simulink library "halin"  (R2021b)
settings: Solver=VariableStepAuto  StartTime=0.0  StopTime=10.0  RelTol=1e-3
undefined symbols (not defined in the file): KHAL_CAN1ABM1E2E_flg, KHAL_CAN1EPB1E2E_flg, KHAL_CAN1EPS1E2E_flg, KHAL_CAN1ESC1E2E_flg, KHAL_CAN1ESC5E2E_flg, KHAL_CAN3BMS1E2E_flg, KHAL_CAN3BMS6E2E_flg, KHAL_CAN3CCU1E2E_flg, KHAL_CAN3CCU2E2E_flg, KHAL_CAN3MCUNF1E2E_flg, KHAL_CAN3MCUNR1E2E_flg, KHAL_CAN3Shifter1E2E_flg, KHAL_CAN3Shifter2E2E_flg, KHAL_CAN6FCM2E2E_flg, KHAL_CAN6FCM4E2E_flg, TRUE
libraries: simulink x645, FVT_lib x212, hcu_lib x59
(part 11 of 23)

== system halin/HAL_IN/CAN3/CCU1 ==
  DT_CAN3_SG_CCU1 : Inport
  0x35 : Constant  Value=0x35
  0xEB : Constant  Value=0xEB
  BitwiseAND{,1..24} (25 alike) : simulink/Logic and Bit Operations/Bitwise Operator  logicop=AND  UseBitMask=on  BitMask=0xFF  BitMaskRealWorld=Stored Integer
  BitwiseOR{,1..2,9..11} (6 alike) : simulink/Logic and Bit Operations/Bitwise Operator  logicop=OR  UseBitMask=off  BitMask=bin2dec('11011001')  BitMaskRealWorld=Stored Integer
  BitwiseOR3 : simulink/Logic and Bit Operations/Bitwise Operator  logicop=OR  UseBitMask=off  NumInputPorts=3  BitMask=bin2dec('11011001')  BitMaskRealWorld=Stored Integer
  BitwiseOR4 : simulink/Logic and Bit Operations/Bitwise Operator  logicop=OR  UseBitMask=off  NumInputPorts=2  BitMask=bin2dec('11011001')  BitMaskRealWorld=Stored Integer
  BitwiseOR5 : simulink/Logic and Bit Operations/Bitwise Operator  logicop=OR  UseBitMask=off  NumInputPorts=3  BitMask=bin2dec('11011001')  BitMaskRealWorld=Stored Integer
  BitwiseOR6 : simulink/Logic and Bit Operations/Bitwise Operator  logicop=OR  UseBitMask=off  NumInputPorts=2  BitMask=bin2dec('11011001')  BitMaskRealWorld=Stored Integer
  BitwiseOR7 : simulink/Logic and Bit Operations/Bitwise Operator  logicop=OR  UseBitMask=off  NumInputPorts=2  BitMask=bin2dec('11011001')  BitMaskRealWorld=Stored Integer
  BitwiseOR8 : simulink/Logic and Bit Operations/Bitwise Operator  logicop=OR  UseBitMask=off  NumInputPorts=7  BitMask=bin2dec('11011001')  BitMaskRealWorld=Stored Integer
  CSCCU1 : Subsystem
  DCDCAuxCur : Subsystem
  DCDCAuxVolt : Subsystem
  DCDCHVCur : Subsystem
  DCDCInVoltInf : Subsystem
  DCDCPreCompleted : Subsystem
  DDM_CS&RC_Comparison : FVT_lib/hal/DDM_CS&RC_Comparison  MsgCycleTime=10
  Data Type Conversion{,1..24} (25 alike) : DataTypeConversion  OutDataTypeStr=uint8
  KHAL_CAN3CCU1E2E_flg : Constant  Value=KHAL_CAN3CCU1E2E_flg
  LeftShift : ArithShift  BitShiftDirection=Left
  LeftShift1 : ArithShift  BitShiftNumber=5  BitShiftDirection=Left
  LeftShift10 : ArithShift  BitShiftDirection=Left
  LeftShift2 : ArithShift  BitShiftNumber=4  BitShiftDirection=Left
  LeftShift3 : ArithShift  BitShiftNumber=5  BitShiftDirection=Left
  LeftShift4 : ArithShift  BitShiftNumber=3  BitShiftDirection=Left
  LeftShift5 : ArithShift  BitShiftNumber=2  BitShiftDirection=Left
  LeftShift6 : ArithShift  BitShiftNumber=6  BitShiftDirection=Left
  LeftShift7 : ArithShift  BitShiftNumber=7  BitShiftDirection=Left
  LeftShift8 : ArithShift  BitShiftDirection=Left
  LeftShift9 : ArithShift  BitShiftNumber=3  BitShiftDirection=Left
  MessageRollingCounter : FVT_lib/hal/MessageRollingCounter  CounterMAX=14  task_time_ms=5  msg_time_ms=10
  Mux : Mux  Inputs=11
  OBCDCCurrInf : Subsystem
  OBCDCVoltInf : Subsystem
  OBCPreCompleted : Subsystem
  OBCWakeup4Plugin : Subsystem
  RCCCU1 : Subsystem
  RightShift : ArithShift  BitShiftNumber=4
  RightShift1 : ArithShift  BitShiftNumber=-4
  RightShift10 : ArithShift  BitShiftNumber=4
  RightShift11 : ArithShift  BitShiftNumber=-4
  RightShift12 : ArithShift  BitShiftNumber=1
  RightShift13 : ArithShift  BitShiftNumber=-7
  RightShift2 : ArithShift  BitShiftNumber=7
  RightShift3 : ArithShift  BitShiftNumber=-1
  RightShift4 : ArithShift  BitShiftNumber=8
  RightShift5 : ArithShift
  RightShift6 : ArithShift  BitShiftNumber=7
  RightShift7 : ArithShift  BitShiftNumber=-1
  RightShift8 : ArithShift  BitShiftNumber=7
  RightShift9 : ArithShift  BitShiftNumber=-1
  bus_selector : BusSelector  OutputSignals=CAN3_CS_CCU1,CAN3_DCDCAuxCur,CAN3_DCDCAuxVolt,CAN3_DCDCHVCur,CAN3_DCDCInVoltInf,CAN3_DCDCPreCompleted,CAN3_OBCDCCurrInf,CAN3_OBCDCVoltInf,CAN3_OBCPreCompleted,CAN3_OBCV2LINVOTP,CAN3_OBCV2LInsuFault,CAN3_OBCV2LVinOVP,CAN3_OBCV2LVinUVP,CAN3_OBCV2LVoutOCP,CAN3_OBCV2LVoutOVP,CAN3_OBCV2LVoutUVP,CAN3_OBCWakeup4Plugin,CAN3_RC_CCU1
  bus_selector1 : BusSelector  OutputSignals=CAN3_CS_CCU1
  bus_selector10 : BusSelector  OutputSignals=CAN3_OBCWakeup4Plugin
  bus_selector11 : BusSelector  OutputSignals=CAN3_RC_CCU1
  bus_selector2 : BusSelector  OutputSignals=CAN3_DCDCAuxCur
  bus_selector3 : BusSelector  OutputSignals=CAN3_DCDCAuxVolt
  bus_selector4 : BusSelector  OutputSignals=CAN3_DCDCHVCur
  bus_selector5 : BusSelector  OutputSignals=CAN3_DCDCInVoltInf
  bus_selector6 : BusSelector  OutputSignals=CAN3_DCDCPreCompleted
  bus_selector7 : BusSelector  OutputSignals=CAN3_OBCDCCurrInf
  bus_selector8 : BusSelector  OutputSignals=CAN3_OBCDCVoltInf
  bus_selector9 : BusSelector  OutputSignals=CAN3_OBCPreCompleted
  VHAL_CCU1CSErr_flg : Outport
  VHAL_CCU1RCErr_flg : Outport  Port=2
  VHAL_CSCCU1_enum : Outport  Port=3
  VHAL_DCDCAuxCur_A : Outport  Port=4
  VHAL_DCDCAuxVolt_V : Outport  Port=5
  VHAL_DCDCHVCur_A : Outport  Port=6
  VHAL_DCDCInVoltInf_V : Outport  Port=7
  VHAL_DCDCPreCompleted_enum : Outport  Port=8
  VHAL_OBCDCCurrInf_A : Outport  Port=9
  VHAL_OBCDCVoltInf_V : Outport  Port=10
  VHAL_OBCPreCompleted_enum : Outport  Port=11
  VHAL_OBCWakeup4Plugin_flg : Outport  Port=12
  VHAL_RCCCU1_enum : Outport  Port=13
  wires:
  DT_CAN3_SG_CCU1/1 -> [DT_CAN3_SG_CCU1]
  [DT_CAN3_SG_CCU1] -> bus_selector/1
  bus_selector/1 -> [CAN3_CS_CCU1]  "<CAN3_CS_CCU1>"
  [CAN3_CS_CCU1] -> LeftShift/1
  LeftShift/1 -> BitwiseAND/1
  BitwiseAND/1 -> [Byte_0_CAN3_CS_CCU1]
  bus_selector/2 -> [CAN3_DCDCAuxCur]  "<CAN3_DCDCAuxCur>"
  [CAN3_DCDCAuxCur] -> RightShift/1, RightShift1/1
  RightShift/1 -> BitwiseAND1/1
  BitwiseAND1/1 -> [Byte_10_CAN3_DCDCAuxCur]
  RightShift1/1 -> BitwiseAND2/1
  BitwiseAND2/1 -> [Byte_11_CAN3_DCDCAuxCur]
  bus_selector/3 -> [CAN3_DCDCAuxVolt]  "<CAN3_DCDCAuxVolt>"
  [CAN3_DCDCAuxVolt] -> RightShift2/1, RightShift3/1
  RightShift2/1 -> BitwiseAND3/1
  BitwiseAND3/1 -> [Byte_6_CAN3_DCDCAuxVolt]
  RightShift3/1 -> BitwiseAND4/1
  BitwiseAND4/1 -> [Byte_7_CAN3_DCDCAuxVolt]
  bus_selector/4 -> [CAN3_DCDCHVCur]  "<CAN3_DCDCHVCur>"
  [CAN3_DCDCHVCur] -> RightShift4/1, RightShift5/1
  RightShift4/1 -> BitwiseAND5/1
  BitwiseAND5/1 -> [Byte_8_CAN3_DCDCHVCur]
  RightShift5/1 -> BitwiseAND6/1
  BitwiseAND6/1 -> [Byte_9_CAN3_DCDCHVCur]
  bus_selector/5 -> [CAN3_DCDCInVoltInf]  "<CAN3_DCDCInVoltInf>"
  [CAN3_DCDCInVoltInf] -> RightShift6/1, RightShift7/1
  RightShift6/1 -> BitwiseAND7/1
  BitwiseAND7/1 -> [Byte_5_CAN3_DCDCInVoltInf]
  RightShift7/1 -> BitwiseAND8/1
  BitwiseAND8/1 -> [Byte_6_CAN3_DCDCInVoltInf]
  bus_selector/6 -> [CAN3_DCDCPreCompleted]  "<CAN3_DCDCPreCompleted>"
  [CAN3_DCDCPreCompleted] -> LeftShift1/1
  LeftShift1/1 -> BitwiseAND9/1
  BitwiseAND9/1 -> [Byte_5_CAN3_DCDCPreCompleted]
  bus_selector/7 -> [CAN3_OBCDCCurrInf]  "<CAN3_OBCDCCurrInf>"
  [CAN3_OBCDCCurrInf] -> RightShift8/1, RightShift9/1
  RightShift8/1 -> BitwiseAND10/1
  BitwiseAND10/1 -> [Byte_3_CAN3_OBCDCCurrInf]
  RightShift9/1 -> BitwiseAND11/1
  BitwiseAND11/1 -> [Byte_4_CAN3_OBCDCCurrInf]
  bus_selector/8 -> [CAN3_OBCDCVoltInf]  "<CAN3_OBCDCVoltInf>"
  [CAN3_OBCDCVoltInf] -> RightShift10/1, RightShift11/1
  RightShift10/1 -> BitwiseAND12/1
  BitwiseAND12/1 -> [Byte_2_CAN3_OBCDCVoltInf]
  RightShift11/1 -> BitwiseAND13/1
  BitwiseAND13/1 -> [Byte_3_CAN3_OBCDCVoltInf]
  bus_selector/9 -> [CAN3_OBCPreCompleted]  "<CAN3_OBCPreCompleted>"
  [CAN3_OBCPreCompleted] -> RightShift12/1, RightShift13/1
  RightShift12/1 -> BitwiseAND14/1
  BitwiseAND14/1 -> [Byte_4_CAN3_OBCPreCompleted]
  RightShift13/1 -> BitwiseAND15/1
  BitwiseAND15/1 -> [Byte_5_CAN3_OBCPreCompleted]
  bus_selector/10 -> [CAN3_OBCV2LINVOTP]  "<CAN3_OBCV2LINVOTP>"
  [CAN3_OBCV2LINVOTP] -> LeftShift2/1
  LeftShift2/1 -> BitwiseAND16/1
  BitwiseAND16/1 -> [Byte_8_CAN3_OBCV2LINVOTP]
  bus_selector/11 -> [CAN3_OBCV2LInsuFault]  "<CAN3_OBCV2LInsuFault>"
  [CAN3_OBCV2LInsuFault] -> LeftShift3/1
  LeftShift3/1 -> BitwiseAND17/1
  BitwiseAND17/1 -> [Byte_8_CAN3_OBCV2LInsuFault]
  bus_selector/12 -> [CAN3_OBCV2LVinOVP]  "<CAN3_OBCV2LVinOVP>"
  [CAN3_OBCV2LVinOVP] -> LeftShift4/1
  LeftShift4/1 -> BitwiseAND18/1
  BitwiseAND18/1 -> [Byte_8_CAN3_OBCV2LVinOVP]
  bus_selector/13 -> [CAN3_OBCV2LVinUVP]  "<CAN3_OBCV2LVinUVP>"
  [CAN3_OBCV2LVinUVP] -> LeftShift5/1
  LeftShift5/1 -> BitwiseAND19/1
  BitwiseAND19/1 -> [Byte_8_CAN3_OBCV2LVinUVP]
  bus_selector/14 -> [CAN3_OBCV2LVoutOCP]  "<CAN3_OBCV2LVoutOCP>"
  [CAN3_OBCV2LVoutOCP] -> LeftShift6/1
  LeftShift6/1 -> BitwiseAND20/1
  BitwiseAND20/1 -> [Byte_8_CAN3_OBCV2LVoutOCP]
  bus_selector/15 -> [CAN3_OBCV2LVoutOVP]  "<CAN3_OBCV2LVoutOVP>"
  [CAN3_OBCV2LVoutOVP] -> LeftShift7/1
  LeftShift7/1 -> BitwiseAND21/1
  BitwiseAND21/1 -> [Byte_8_CAN3_OBCV2LVoutOVP]
  bus_selector/16 -> [CAN3_OBCV2LVoutUVP]  "<CAN3_OBCV2LVoutUVP>"
  [CAN3_OBCV2LVoutUVP] -> LeftShift8/1
  LeftShift8/1 -> BitwiseAND22/1
  BitwiseAND22/1 -> [Byte_7_CAN3_OBCV2LVoutUVP]
  bus_selector/17 -> [CAN3_OBCWakeup4Plugin]  "<CAN3_OBCWakeup4Plugin>"
  [CAN3_OBCWakeup4Plugin] -> LeftShift9/1
  LeftShift9/1 -> BitwiseAND23/1
  BitwiseAND23/1 -> [Byte_3_CAN3_OBCWakeup4Plugin]
  bus_selector/18 -> [CAN3_RC_CCU1]  "<CAN3_RC_CCU1>"
  [CAN3_RC_CCU1] -> LeftShift10/1
  LeftShift10/1 -> BitwiseAND24/1
  BitwiseAND24/1 -> [Byte_1_CAN3_RC_CCU1]
  Data Type Conversion/1 -> BitwiseOR/1
  [Byte_0_CAN3_CS_CCU1] -> Data Type Conversion/1
  BitwiseOR/1 -> [Byte_0]
  Data Type Conversion1/1 -> BitwiseOR1/1
  [Byte_1_CAN3_RC_CCU1] -> Data Type Conversion1/1
  BitwiseOR1/1 -> [Byte_1]
  Data Type Conversion2/1 -> BitwiseOR2/1
  [Byte_2_CAN3_OBCDCVoltInf] -> Data Type Conversion2/1
  BitwiseOR2/1 -> [Byte_2]
  Data Type Conversion3/1 -> BitwiseOR3/1
  [Byte_3_CAN3_OBCDCCurrInf] -> Data Type Conversion3/1
  Data Type Conversion4/1 -> BitwiseOR3/2
  [Byte_3_CAN3_OBCDCVoltInf] -> Data Type Conversion4/1
  Data Type Conversion5/1 -> BitwiseOR3/3
  [Byte_3_CAN3_OBCWakeup4Plugin] -> Data Type Conversion5/1
  BitwiseOR3/1 -> [Byte_3]
  Data Type Conversion6/1 -> BitwiseOR4/1
  [Byte_4_CAN3_OBCDCCurrInf] -> Data Type Conversion6/1
  Data Type Conversion7/1 -> BitwiseOR4/2
  [Byte_4_CAN3_OBCPreCompleted] -> Data Type Conversion7/1
  BitwiseOR4/1 -> [Byte_4]
  Data Type Conversion8/1 -> BitwiseOR5/1
  [Byte_5_CAN3_DCDCInVoltInf] -> Data Type Conversion8/1
  Data Type Conversion9/1 -> BitwiseOR5/2
  [Byte_5_CAN3_DCDCPreCompleted] -> Data Type Conversion9/1
  Data Type Conversion10/1 -> BitwiseOR5/3
  [Byte_5_CAN3_OBCPreCompleted] -> Data Type Conversion10/1
  BitwiseOR5/1 -> [Byte_5]
  Data Type Conversion11/1 -> BitwiseOR6/1
  [Byte_6_CAN3_DCDCAuxVolt] -> Data Type Conversion11/1
  Data Type Conversion12/1 -> BitwiseOR6/2
  [Byte_6_CAN3_DCDCInVoltInf] -> Data Type Conversion12/1
  BitwiseOR6/1 -> [Byte_6]
  Data Type Conversion13/1 -> BitwiseOR7/1
  [Byte_7_CAN3_DCDCAuxVolt] -> Data Type Conversion13/1
  Data Type Conversion14/1 -> BitwiseOR7/2
  [Byte_7_CAN3_OBCV2LVoutUVP] -> Data Type Conversion14/1
  BitwiseOR7/1 -> [Byte_7]
  Data Type Conversion15/1 -> BitwiseOR8/1
  [Byte_8_CAN3_DCDCHVCur] -> Data Type Conversion15/1
  Data Type Conversion16/1 -> BitwiseOR8/2
  [Byte_8_CAN3_OBCV2LINVOTP] -> Data Type Conversion16/1
  Data Type Conversion17/1 -> BitwiseOR8/3
  [Byte_8_CAN3_OBCV2LInsuFault] -> Data Type Conversion17/1
  Data Type Conversion18/1 -> BitwiseOR8/4
  [Byte_8_CAN3_OBCV2LVinOVP] -> Data Type Conversion18/1
  Data Type Conversion19/1 -> BitwiseOR8/5
  [Byte_8_CAN3_OBCV2LVinUVP] -> Data Type Conversion19/1
  Data Type Conversion20/1 -> BitwiseOR8/6
  [Byte_8_CAN3_OBCV2LVoutOCP] -> Data Type Conversion20/1
  Data Type Conversion21/1 -> BitwiseOR8/7
  [Byte_8_CAN3_OBCV2LVoutOVP] -> Data Type Conversion21/1
  BitwiseOR8/1 -> [Byte_8]
  Data Type Conversion22/1 -> BitwiseOR9/1
  [Byte_9_CAN3_DCDCHVCur] -> Data Type Conversion22/1
  BitwiseOR9/1 -> [Byte_9]
  Data Type Conversion23/1 -> BitwiseOR10/1
  [Byte_10_CAN3_DCDCAuxCur] -> Data Type Conversion23/1
  BitwiseOR10/1 -> [Byte_10]
  Data Type Conversion24/1 -> BitwiseOR11/1
  [Byte_11_CAN3_DCDCAuxCur] -> Data Type Conversion24/1
  BitwiseOR11/1 -> [Byte_11]
  [Byte_1] -> Mux/1
  [Byte_2] -> Mux/2
  [Byte_3] -> Mux/3
  [Byte_4] -> Mux/4
  [Byte_5] -> Mux/5
  [Byte_6] -> Mux/6
  [Byte_7] -> Mux/7
  [Byte_8] -> Mux/8
  [Byte_9] -> Mux/9
  [Byte_10] -> Mux/10
  [Byte_11] -> Mux/11
  Mux/1 -> [VHAL_CAN3CCU1noCS_raw]
  KHAL_CAN3CCU1E2E_flg/1 -> DDM_CS&RC_Comparison/1
  0x35/1 -> DDM_CS&RC_Comparison/2
  0xEB/1 -> DDM_CS&RC_Comparison/3
  [VHAL_CAN3CCU1noCS_raw] -> DDM_CS&RC_Comparison/4
  [Byte_0] -> DDM_CS&RC_Comparison/5
  [RC_ECU] -> DDM_CS&RC_Comparison/6
  MessageRollingCounter/1 -> DDM_CS&RC_Comparison/7
  DDM_CS&RC_Comparison/1 -> VHAL_CCU1CSErr_flg/1
  DDM_CS&RC_Comparison/2 -> VHAL_CCU1RCErr_flg/1
  [DT_CAN3_SG_CCU1] -> bus_selector1/1
  bus_selector1/1 -> CSCCU1/1(CS_CCU1)  "<CAN3_CS_CCU1>"
  CSCCU1/1(VHAL_CSCCU1_enum) -> VHAL_CSCCU1_enum/1
  [DT_CAN3_SG_CCU1] -> bus_selector2/1
  bus_selector2/1 -> DCDCAuxCur/1(DCDCAuxCur)  "<CAN3_DCDCAuxCur>"
  DCDCAuxCur/1(VHAL_DCDCAuxCur_A) -> VHAL_DCDCAuxCur_A/1
  [DT_CAN3_SG_CCU1] -> bus_selector3/1
  bus_selector3/1 -> DCDCAuxVolt/1(DCDCAuxVolt)  "<CAN3_DCDCAuxVolt>"
  DCDCAuxVolt/1(VHAL_DCDCAuxVolt_V) -> VHAL_DCDCAuxVolt_V/1
  [DT_CAN3_SG_CCU1] -> bus_selector4/1
  bus_selector4/1 -> DCDCHVCur/1(DCDCHVCur)  "<CAN3_DCDCHVCur>"
  DCDCHVCur/1(VHAL_DCDCHVCur_A) -> VHAL_DCDCHVCur_A/1
  [DT_CAN3_SG_CCU1] -> bus_selector5/1
  bus_selector5/1 -> DCDCInVoltInf/1(DCDCInVoltInf)  "<CAN3_DCDCInVoltInf>"
  DCDCInVoltInf/1(VHAL_DCDCInVoltInf_V) -> VHAL_DCDCInVoltInf_V/1
  [DT_CAN3_SG_CCU1] -> bus_selector6/1
  bus_selector6/1 -> DCDCPreCompleted/1(DCDCPreCompleted)  "<CAN3_DCDCPreCompleted>"
  DCDCPreCompleted/1(VHAL_DCDCPreCompleted_enum) -> VHAL_DCDCPreCompleted_enum/1
  [DT_CAN3_SG_CCU1] -> bus_selector7/1
  bus_selector7/1 -> OBCDCCurrInf/1(OBCDCCurrInf)  "<CAN3_OBCDCCurrInf>"
  OBCDCCurrInf/1(VHAL_OBCDCCurrInf_A) -> VHAL_OBCDCCurrInf_A/1
  [DT_CAN3_SG_CCU1] -> bus_selector8/1
  bus_selector8/1 -> OBCDCVoltInf/1(OBCDCVoltInf)  "<CAN3_OBCDCVoltInf>"
  OBCDCVoltInf/1(VHAL_OBCDCVoltInf_V) -> VHAL_OBCDCVoltInf_V/1
  [DT_CAN3_SG_CCU1] -> bus_selector9/1
  bus_selector9/1 -> OBCPreCompleted/1(OBCPreCompleted)  "<CAN3_OBCPreCompleted>"
  OBCPreCompleted/1(VHAL_OBCPreCompleted_enum) -> VHAL_OBCPreCompleted_enum/1
  [DT_CAN3_SG_CCU1] -> bus_selector10/1
  bus_selector10/1 -> OBCWakeup4Plugin/1(OBCWakeup4Plugin)  "<CAN3_OBCWakeup4Plugin>"
  OBCWakeup4Plugin/1(VHAL_OBCWakeup4Plugin_flg) -> VHAL_OBCWakeup4Plugin_flg/1
  [DT_CAN3_SG_CCU1] -> bus_selector11/1
  bus_selector11/1 -> RCCCU1/1(RC_CCU1)  "<CAN3_RC_CCU1>"
  RCCCU1/1(VHAL_RCCCU1_enum) -> VHAL_RCCCU1_enum/1, [RC_ECU]

== system halin/HAL_IN/CAN3/CCU2 ==
  DT_CAN3_SG_CCU2 : Inport
  0x21 : Constant  Value=0x21
  0xE6 : Constant  Value=0xE6
  BitwiseAND{,1..20} (21 alike) : simulink/Logic and Bit Operations/Bitwise Operator  logicop=AND  UseBitMask=on  BitMask=0xFF  BitMaskRealWorld=Stored Integer
  BitwiseOR{,1..2,4..5,7..9} (8 alike) : simulink/Logic and Bit Operations/Bitwise Operator  logicop=OR  UseBitMask=off  BitMask=bin2dec('11011001')  BitMaskRealWorld=Stored Integer
  BitwiseOR10 : simulink/Logic and Bit Operations/Bitwise Operator  logicop=OR  UseBitMask=off  NumInputPorts=5  BitMask=bin2dec('11011001')  BitMaskRealWorld=Stored Integer
  BitwiseOR3 : simulink/Logic and Bit Operations/Bitwise Operator  logicop=OR  UseBitMask=off  NumInputPorts=3  BitMask=bin2dec('11011001')  BitMaskRealWorld=Stored Integer
  BitwiseOR6 : simulink/Logic and Bit Operations/Bitwise Operator  logicop=OR  UseBitMask=off  NumInputPorts=5  BitMask=bin2dec('11011001')  BitMaskRealWorld=Stored Integer
  CSCCU2 : Subsystem
  DCDCEnaSta : Subsystem
  DCDCFaultSta : Subsystem
  DCDCReady4Pre : Subsystem
  DCDCTemp : Subsystem
  DDM_CS&RC_Comparison : FVT_lib/hal/DDM_CS&RC_Comparison  MsgCycleTime=100
  Data Type Conversion{,1..20} (21 alike) : DataTypeConversion  OutDataTypeStr=uint8
  KHAL_CAN3CCU2E2E_flg : Constant  Value=KHAL_CAN3CCU2E2E_flg
  LeftShift{,4,6,12} (4 alike) : ArithShift  BitShiftDirection=Left
  LeftShift1 : ArithShift  BitShiftNumber=2  BitShiftDirection=Left
  LeftShift10 : ArithShift  BitShiftNumber=6  BitShiftDirection=Left
  LeftShift11 : ArithShift  BitShiftNumber=4  BitShiftDirection=Left
  LeftShift2 : ArithShift  BitShiftNumber=2  BitShiftDirection=Left
  LeftShift3 : ArithShift  BitShiftNumber=5  BitShiftDirection=Left
  LeftShift5 : ArithShift  BitShiftNumber=4  BitShiftDirection=Left
  LeftShift7 : ArithShift  BitShiftNumber=3  BitShiftDirection=Left
  LeftShift8 : ArithShift  BitShiftNumber=4  BitShiftDirection=Left
  LeftShift9 : ArithShift  BitShiftNumber=6  BitShiftDirection=Left
  MessageRollingCounter : FVT_lib/hal/MessageRollingCounter  CounterMAX=14  task_time_ms=5  msg_time_ms=100
  Mux : Mux  Inputs=11
  OBCACCurLim : Subsystem
  OBCACCurrInf : Subsystem
  OBCACVoltInf : Subsystem
  OBCEnaSta : Subsystem
  OBCFaultSta : Subsystem
  OBCPluginSta : Subsystem
  OBCReady4Pre : Subsystem
  OBCTemp : Subsystem
  OBCV2LSta : Subsystem
  RCCCU2 : Subsystem
  RightShift : ArithShift  BitShiftNumber=2
  RightShift1 : ArithShift  BitShiftNumber=-6
  RightShift2 : ArithShift  BitShiftNumber=8
  RightShift3 : ArithShift
  RightShift4 : ArithShift  BitShiftNumber=8
  RightShift5 : ArithShift
  RightShift6 : ArithShift  BitShiftNumber=1
  RightShift7 : ArithShift  BitShiftNumber=-7
  bus_selector : BusSelector  OutputSignals=CAN3_CS_CCU2,CAN3_DCDCEnaSta,CAN3_DCDCFaultSta,CAN3_DCDCReady4Pre,CAN3_DCDCTemp,CAN3_OBCACCurrInf,CAN3_OBCACVoltInf,CAN3_OBCDCP,CAN3_OBCEnaSta,CAN3_OBCFaultSta,CAN3_OBCPluginSta,CAN3_OBCReady4Pre,CAN3_OBCRlySta,CAN3_OBCTemp,CAN3_OBCV2LSta,CAN3_OBC_AC_Cur_Lim,CAN3_RC_CCU2
  bus_selector1 : BusSelector  OutputSignals=CAN3_CS_CCU2
  bus_selector10 : BusSelector  OutputSignals=CAN3_OBCPluginSta
  bus_selector11 : BusSelector  OutputSignals=CAN3_OBCReady4Pre
  bus_selector12 : BusSelector  OutputSignals=CAN3_OBCTemp
  bus_selector13 : BusSelector  OutputSignals=CAN3_OBCV2LSta
  bus_selector14 : BusSelector  OutputSignals=CAN3_OBC_AC_Cur_Lim
  bus_selector15 : BusSelector  OutputSignals=CAN3_RC_CCU2
  bus_selector2 : BusSelector  OutputSignals=CAN3_DCDCEnaSta
  bus_selector3 : BusSelector  OutputSignals=CAN3_DCDCFaultSta
  bus_selector4 : BusSelector  OutputSignals=CAN3_DCDCReady4Pre
  bus_selector5 : BusSelector  OutputSignals=CAN3_DCDCTemp
  bus_selector6 : BusSelector  OutputSignals=CAN3_OBCACCurrInf
  bus_selector7 : BusSelector  OutputSignals=CAN3_OBCACVoltInf
  bus_selector8 : BusSelector  OutputSignals=CAN3_OBCEnaSta
  bus_selector9 : BusSelector  OutputSignals=CAN3_OBCFaultSta
  constant : Constant  Value=0x0  OutDataTypeStr=uint8
  VHAL_CCU2CSErr_flg : Outport
  VHAL_CCU2RCErr_flg : Outport  Port=2
  VHAL_CSCCU2_enum : Outport  Port=3
  VHAL_DCDCEnaSta_flg : Outport  Port=4
  VHAL_DCDCFaultSta_enum : Outport  Port=5
  VHAL_DCDCReady4Pre_flg : Outport  Port=6
  VHAL_DCDCTemp_C : Outport  Port=7
  VHAL_OBCACCurrInf_A : Outport  Port=8
  VHAL_OBCACVoltInf_V : Outport  Port=9
  VHAL_OBCEnaSta_flg : Outport  Port=10
  VHAL_OBCFaultSta_enum : Outport  Port=11
  VHAL_OBCPluginSta_flg : Outport  Port=12
  VHAL_OBCReady4Pre_flg : Outport  Port=13
  VHAL_OBCTemp_C : Outport  Port=14
  VHAL_OBCV2LSta_enum : Outport  Port=15
  VHAL_OBCACCurLim_enum : Outport  Port=16
  VHAL_RCCCU2_enum : Outport  Port=17
  wires:
  DT_CAN3_SG_CCU2/1 -> [DT_CAN3_SG_CCU2]
  [DT_CAN3_SG_CCU2] -> bus_selector/1
  bus_selector/1 -> [CAN3_CS_CCU2]  "<CAN3_CS_CCU2>"
  [CAN3_CS_CCU2] -> LeftShift/1
  LeftShift/1 -> BitwiseAND/1
  BitwiseAND/1 -> [Byte_0_CAN3_CS_CCU2]
  bus_selector/2 -> [CAN3_DCDCEnaSta]  "<CAN3_DCDCEnaSta>"
  [CAN3_DCDCEnaSta] -> LeftShift1/1
  LeftShift1/1 -> BitwiseAND1/1
  BitwiseAND1/1 -> [Byte_7_CAN3_DCDCEnaSta]
  bus_selector/3 -> [CAN3_DCDCFaultSta]  "<CAN3_DCDCFaultSta>"
  [CAN3_DCDCFaultSta] -> LeftShift2/1
  LeftShift2/1 -> BitwiseAND2/1
  BitwiseAND2/1 -> [Byte_11_CAN3_DCDCFaultSta]
  bus_selector/4 -> [CAN3_DCDCReady4Pre]  "<CAN3_DCDCReady4Pre>"
  [CAN3_DCDCReady4Pre] -> LeftShift3/1
  LeftShift3/1 -> BitwiseAND3/1
  BitwiseAND3/1 -> [Byte_11_CAN3_DCDCReady4Pre]
  bus_selector/5 -> [CAN3_DCDCTemp]  "<CAN3_DCDCTemp>"
  [CAN3_DCDCTemp] -> LeftShift4/1
  LeftShift4/1 -> BitwiseAND4/1
  BitwiseAND4/1 -> [Byte_9_CAN3_DCDCTemp]
  bus_selector/6 -> [CAN3_OBCACCurrInf]  "<CAN3_OBCACCurrInf>"
  [CAN3_OBCACCurrInf] -> RightShift/1, RightShift1/1
  RightShift/1 -> BitwiseAND5/1
  BitwiseAND5/1 -> [Byte_6_CAN3_OBCACCurrInf]
  RightShift1/1 -> BitwiseAND6/1
  BitwiseAND6/1 -> [Byte_7_CAN3_OBCACCurrInf]
  bus_selector/7 -> [CAN3_OBCACVoltInf]  "<CAN3_OBCACVoltInf>"
  [CAN3_OBCACVoltInf] -> RightShift2/1, RightShift3/1
  RightShift2/1 -> BitwiseAND7/1
  BitwiseAND7/1 -> [Byte_4_CAN3_OBCACVoltInf]
  RightShift3/1 -> BitwiseAND8/1
  BitwiseAND8/1 -> [Byte_5_CAN3_OBCACVoltInf]
  bus_selector/8 -> [CAN3_OBCDCP]  "<CAN3_OBCDCP>"
  [CAN3_OBCDCP] -> RightShift4/1, RightShift5/1
  RightShift4/1 -> BitwiseAND9/1
  BitwiseAND9/1 -> [Byte_7_CAN3_OBCDCP]
  RightShift5/1 -> BitwiseAND10/1
  BitwiseAND10/1 -> [Byte_8_CAN3_OBCDCP]
  bus_selector/9 -> [CAN3_OBCEnaSta]  "<CAN3_OBCEnaSta>"
  [CAN3_OBCEnaSta] -> LeftShift5/1
  LeftShift5/1 -> BitwiseAND11/1
  BitwiseAND11/1 -> [Byte_7_CAN3_OBCEnaSta]
  bus_selector/10 -> [CAN3_OBCFaultSta]  "<CAN3_OBCFaultSta>"
  [CAN3_OBCFaultSta] -> LeftShift6/1
  LeftShift6/1 -> BitwiseAND12/1
  BitwiseAND12/1 -> [Byte_11_CAN3_OBCFaultSta]
  bus_selector/11 -> [CAN3_OBCPluginSta]  "<CAN3_OBCPluginSta>"
  [CAN3_OBCPluginSta] -> LeftShift7/1
  LeftShift7/1 -> BitwiseAND13/1
  BitwiseAND13/1 -> [Byte_7_CAN3_OBCPluginSta]
  bus_selector/12 -> [CAN3_OBCReady4Pre]  "<CAN3_OBCReady4Pre>"
  [CAN3_OBCReady4Pre] -> LeftShift8/1
  LeftShift8/1 -> BitwiseAND14/1
  BitwiseAND14/1 -> [Byte_11_CAN3_OBCReady4Pre]
  bus_selector/13 -> [CAN3_OBCRlySta]  "<CAN3_OBCRlySta>"
  [CAN3_OBCRlySta] -> LeftShift9/1
  LeftShift9/1 -> BitwiseAND15/1
  BitwiseAND15/1 -> [Byte_4_CAN3_OBCRlySta]
  bus_selector/14 -> [CAN3_OBCTemp]  "<CAN3_OBCTemp>"
  [CAN3_OBCTemp] -> RightShift6/1, RightShift7/1
  RightShift6/1 -> BitwiseAND16/1
  BitwiseAND16/1 -> [Byte_10_CAN3_OBCTemp]
  RightShift7/1 -> BitwiseAND17/1
  BitwiseAND17/1 -> [Byte_11_CAN3_OBCTemp]
  bus_selector/15 -> [CAN3_OBCV2LSta]  "<CAN3_OBCV2LSta>"
  [CAN3_OBCV2LSta] -> LeftShift10/1
  LeftShift10/1 -> BitwiseAND18/1
  BitwiseAND18/1 -> [Byte_3_CAN3_OBCV2LSta]
  bus_selector/16 -> [CAN3_OBC_AC_Cur_Lim]  "<CAN3_OBC_AC_Cur_Lim>"
  [CAN3_OBC_AC_Cur_Lim] -> LeftShift11/1
  LeftShift11/1 -> BitwiseAND19/1
  BitwiseAND19/1 -> [Byte_4_CAN3_OBC_AC_Cur_Lim]
  bus_selector/17 -> [CAN3_RC_CCU2]  "<CAN3_RC_CCU2>"
  [CAN3_RC_CCU2] -> LeftShift12/1
  LeftShift12/1 -> BitwiseAND20/1
  BitwiseAND20/1 -> [Byte_1_CAN3_RC_CCU2]
  Data Type Conversion/1 -> BitwiseOR/1
  [Byte_0_CAN3_CS_CCU2] -> Data Type Conversion/1
  BitwiseOR/1 -> [Byte_0]
  Data Type Conversion1/1 -> BitwiseOR1/1
  [Byte_1_CAN3_RC_CCU2] -> Data Type Conversion1/1
  BitwiseOR1/1 -> [Byte_1]
  constant/1 -> [Byte_2]
  Data Type Conversion2/1 -> BitwiseOR2/1
  [Byte_3_CAN3_OBCV2LSta] -> Data Type Conversion2/1
  BitwiseOR2/1 -> [Byte_3]
  Data Type Conversion3/1 -> BitwiseOR3/1
  [Byte_4_CAN3_OBCACVoltInf] -> Data Type Conversion3/1
  Data Type Conversion4/1 -> BitwiseOR3/2
  [Byte_4_CAN3_OBCRlySta] -> Data Type Conversion4/1
  Data Type Conversion5/1 -> BitwiseOR3/3
  [Byte_4_CAN3_OBC_AC_Cur_Lim] -> Data Type Conversion5/1
  BitwiseOR3/1 -> [Byte_4]
  Data Type Conversion6/1 -> BitwiseOR4/1
  [Byte_5_CAN3_OBCACVoltInf] -> Data Type Conversion6/1
  BitwiseOR4/1 -> [Byte_5]
  Data Type Conversion7/1 -> BitwiseOR5/1
  [Byte_6_CAN3_OBCACCurrInf] -> Data Type Conversion7/1
  BitwiseOR5/1 -> [Byte_6]
  Data Type Conversion8/1 -> BitwiseOR6/1
  [Byte_7_CAN3_DCDCEnaSta] -> Data Type Conversion8/1
  Data Type Conversion9/1 -> BitwiseOR6/2
  [Byte_7_CAN3_OBCACCurrInf] -> Data Type Conversion9/1
  Data Type Conversion10/1 -> BitwiseOR6/3
  [Byte_7_CAN3_OBCDCP] -> Data Type Conversion10/1
  Data Type Conversion11/1 -> BitwiseOR6/4
  [Byte_7_CAN3_OBCEnaSta] -> Data Type Conversion11/1
  Data Type Conversion12/1 -> BitwiseOR6/5
  [Byte_7_CAN3_OBCPluginSta] -> Data Type Conversion12/1
  BitwiseOR6/1 -> [Byte_7]
  Data Type Conversion13/1 -> BitwiseOR7/1
  [Byte_8_CAN3_OBCDCP] -> Data Type Conversion13/1
  BitwiseOR7/1 -> [Byte_8]
  Data Type Conversion14/1 -> BitwiseOR8/1
  [Byte_9_CAN3_DCDCTemp] -> Data Type Conversion14/1
  BitwiseOR8/1 -> [Byte_9]
  Data Type Conversion15/1 -> BitwiseOR9/1
  [Byte_10_CAN3_OBCTemp] -> Data Type Conversion15/1
  BitwiseOR9/1 -> [Byte_10]
  Data Type Conversion16/1 -> BitwiseOR10/1
  [Byte_11_CAN3_DCDCFaultSta] -> Data Type Conversion16/1
  Data Type Conversion17/1 -> BitwiseOR10/2
  [Byte_11_CAN3_DCDCReady4Pre] -> Data Type Conversion17/1
  Data Type Conversion18/1 -> BitwiseOR10/3
  [Byte_11_CAN3_OBCFaultSta] -> Data Type Conversion18/1
  Data Type Conversion19/1 -> BitwiseOR10/4
  [Byte_11_CAN3_OBCReady4Pre] -> Data Type Conversion19/1
  Data Type Conversion20/1 -> BitwiseOR10/5
  [Byte_11_CAN3_OBCTemp] -> Data Type Conversion20/1
  BitwiseOR10/1 -> [Byte_11]
  [Byte_1] -> Mux/1
  [Byte_2] -> Mux/2
  [Byte_3] -> Mux/3
  [Byte_4] -> Mux/4
  [Byte_5] -> Mux/5
  [Byte_6] -> Mux/6
  [Byte_7] -> Mux/7
  [Byte_8] -> Mux/8
  [Byte_9] -> Mux/9
  [Byte_10] -> Mux/10
  [Byte_11] -> Mux/11
  Mux/1 -> [VHAL_CAN3CCU2noCS_raw]
  KHAL_CAN3CCU2E2E_flg/1 -> DDM_CS&RC_Comparison/1
  0x21/1 -> DDM_CS&RC_Comparison/2
  0xE6/1 -> DDM_CS&RC_Comparison/3
  [VHAL_CAN3CCU2noCS_raw] -> DDM_CS&RC_Comparison/4
  [Byte_0] -> DDM_CS&RC_Comparison/5
  [RC_ECU] -> DDM_CS&RC_Comparison/6
  MessageRollingCounter/1 -> DDM_CS&RC_Comparison/7
  DDM_CS&RC_Comparison/1 -> VHAL_CCU2CSErr_flg/1
  DDM_CS&RC_Comparison/2 -> VHAL_CCU2RCErr_flg/1
  [DT_CAN3_SG_CCU2] -> bus_selector1/1
  bus_selector1/1 -> CSCCU2/1(CS_CCU2)  "<CAN3_CS_CCU2>"
  CSCCU2/1(VHAL_CSCCU2_enum) -> VHAL_CSCCU2_enum/1
  [DT_CAN3_SG_CCU2] -> bus_selector2/1
  bus_selector2/1 -> DCDCEnaSta/1(DCDCEnaSta)  "<CAN3_DCDCEnaSta>"
  DCDCEnaSta/1(VHAL_DCDCEnaSta_flg) -> VHAL_DCDCEnaSta_flg/1
  [DT_CAN3_SG_CCU2] -> bus_selector3/1
  bus_selector3/1 -> DCDCFaultSta/1(DCDCFaultSta)  "<CAN3_DCDCFaultSta>"
  DCDCFaultSta/1(VHAL_DCDCFaultSta_enum) -> VHAL_DCDCFaultSta_enum/1
  [DT_CAN3_SG_CCU2] -> bus_selector4/1
  bus_selector4/1 -> DCDCReady4Pre/1(DCDCReady4Pre)  "<CAN3_DCDCReady4Pre>"
  DCDCReady4Pre/1(VHAL_DCDCReady4Pre_flg) -> VHAL_DCDCReady4Pre_flg/1
  [DT_CAN3_SG_CCU2] -> bus_selector5/1
  bus_selector5/1 -> DCDCTemp/1(DCDCTemp)  "<CAN3_DCDCTemp>"
  DCDCTemp/1(VHAL_DCDCTemp_C) -> VHAL_DCDCTemp_C/1
  [DT_CAN3_SG_CCU2] -> bus_selector6/1
  bus_selector6/1 -> OBCACCurrInf/1(OBCACCurrInf)  "<CAN3_OBCACCurrInf>"
  OBCACCurrInf/1(VHAL_OBCACCurrInf_A) -> VHAL_OBCACCurrInf_A/1
  [DT_CAN3_SG_CCU2] -> bus_selector7/1
  bus_selector7/1 -> OBCACVoltInf/1(OBCACVoltInf)  "<CAN3_OBCACVoltInf>"
  OBCACVoltInf/1(VHAL_OBCACVoltInf_V) -> VHAL_OBCACVoltInf_V/1
  [DT_CAN3_SG_CCU2] -> bus_selector8/1
  bus_selector8/1 -> OBCEnaSta/1(OBCEnaSta)  "<CAN3_OBCEnaSta>"
  OBCEnaSta/1(VHAL_OBCEnaSta_flg) -> VHAL_OBCEnaSta_flg/1
  [DT_CAN3_SG_CCU2] -> bus_selector9/1
  bus_selector9/1 -> OBCFaultSta/1(OBCFaultSta)  "<CAN3_OBCFaultSta>"
  OBCFaultSta/1(VHAL_OBCFaultSta_enum) -> VHAL_OBCFaultSta_enum/1
  [DT_CAN3_SG_CCU2] -> bus_selector10/1
  bus_selector10/1 -> OBCPluginSta/1(OBCPluginSta)  "<CAN3_OBCPluginSta>"
  OBCPluginSta/1(VHAL_OBCPluginSta_flg) -> VHAL_OBCPluginSta_flg/1
  [DT_CAN3_SG_CCU2] -> bus_selector11/1
  bus_selector11/1 -> OBCReady4Pre/1(OBCReady4Pre)  "<CAN3_OBCReady4Pre>"
  OBCReady4Pre/1(VHAL_OBCReady4Pre_flg) -> VHAL_OBCReady4Pre_flg/1
  [DT_CAN3_SG_CCU2] -> bus_selector12/1
  bus_selector12/1 -> OBCTemp/1(OBCTemp)  "<CAN3_OBCTemp>"
  OBCTemp/1(VHAL_OBCTemp_C) -> VHAL_OBCTemp_C/1
  [DT_CAN3_SG_CCU2] -> bus_selector13/1
  bus_selector13/1 -> OBCV2LSta/1(OBCV2LSta)  "<CAN3_OBCV2LSta>"
  OBCV2LSta/1(VHAL_OBCV2LSta_enum) -> VHAL_OBCV2LSta_enum/1
  [DT_CAN3_SG_CCU2] -> bus_selector14/1
  bus_selector14/1 -> OBCACCurLim/1(OBC_AC_Cur_Lim)  "<CAN3_OBC_AC_Cur_Lim>"
  OBCACCurLim/1(VHAL_OBCACCurLim_enum) -> VHAL_OBCACCurLim_enum/1
  [DT_CAN3_SG_CCU2] -> bus_selector15/1
  bus_selector15/1 -> RCCCU2/1(RC_CCU2)  "<CAN3_RC_CCU2>"
  RCCCU2/1(VHAL_RCCCU2_enum) -> VHAL_RCCCU2_enum/1, [RC_ECU]

== system halin/HAL_IN/CAN3/EBM1 ==
  DT_CAN3_SG_EBM1 : Inport
  EBMErrSta : Subsystem
  EBMRLampSta : Subsystem
  bus_selector : BusSelector  OutputSignals=CAN3_EBMErrSta
  bus_selector1 : BusSelector  OutputSignals=CAN3_EBMRLampSta
  VHAL_EBMErrSta_enum : Outport
  VHAL_EBMRLampSta_enum : Outport  Port=2
  wires:
  DT_CAN3_SG_EBM1/1 -> [DT_CAN3_SG_EBM1]
  [DT_CAN3_SG_EBM1] -> bus_selector/1
  bus_selector/1 -> EBMErrSta/1(EBMErrSta)  "<CAN3_EBMErrSta>"
  EBMErrSta/1(VHAL_EBMErrSta_enum) -> VHAL_EBMErrSta_enum/1
  [DT_CAN3_SG_EBM1] -> bus_selector1/1
  bus_selector1/1 -> EBMRLampSta/1(EBMRLampSta)  "<CAN3_EBMRLampSta>"
  EBMRLampSta/1(VHAL_EBMRLampSta_enum) -> VHAL_EBMRLampSta_enum/1

== system halin/HAL_IN/CAN3/MCU_B_F1 ==
  DT_CAN3_SG_MCU_B_F1 : Inport
  FrActvDmpDisabSta : Subsystem
  FrEDUDrtSta : Subsystem
  FrEDUOpratingSta : Subsystem
  FrEDURealTMTq : Subsystem
  FrEDURotateDirction : Subsystem
  FrEDUTqReqFbk : Subsystem
  FrMCUBAT : Subsystem
  FrMCUDCBusCurr : Subsystem
  FrMCUDCBusVolt : Subsystem
  FrMCUDischrgSta : Subsystem
  FrMCUEnaSta : Subsystem
  FrMCUErr : Subsystem
  FrMCUIGNsta : Subsystem
  FrMCUReady : Subsystem
  FrMCUReady4Pre : Subsystem
  FrMCUSysSta : Subsystem
  FrMCUTemp : Subsystem
  FrMotorAvailTq : Subsystem
  FrRegenAvailTq : Subsystem
  FrTMSpd : Subsystem
  FrTMTemp : Subsystem
  FrTMid : Subsystem
  FrTMiq : Subsystem
  MCUBFRealPwrKwSta : Subsystem
  MCUWarnF : Subsystem
  bus_selector : BusSelector  OutputSignals=CAN3_Fr_ActvDmpDisabSta
  bus_selector1 : BusSelector  OutputSignals=CAN3_Fr_EDUDrtSta
  bus_selector10 : BusSelector  OutputSignals=CAN3_Fr_MCUEnaSta
  bus_selector11 : BusSelector  OutputSignals=CAN3_Fr_MCUErr
  bus_selector12 : BusSelector  OutputSignals=CAN3_Fr_MCUIGN_sta
  bus_selector13 : BusSelector  OutputSignals=CAN3_Fr_MCUReady
  bus_selector14 : BusSelector  OutputSignals=CAN3_Fr_MCUReady4Pre
  bus_selector15 : BusSelector  OutputSignals=CAN3_Fr_MCUSysSta
  bus_selector16 : BusSelector  OutputSignals=CAN3_Fr_MCUTemp
  bus_selector17 : BusSelector  OutputSignals=CAN3_Fr_MotorAvailTq
  bus_selector18 : BusSelector  OutputSignals=CAN3_Fr_RegenAvailTq
  bus_selector19 : BusSelector  OutputSignals=CAN3_Fr_TMSpd
  bus_selector2 : BusSelector  OutputSignals=CAN3_Fr_EDUOpratingSta
  bus_selector20 : BusSelector  OutputSignals=CAN3_Fr_TMTemp
  bus_selector21 : BusSelector  OutputSignals=CAN3_Fr_TMid
  bus_selector22 : BusSelector  OutputSignals=CAN3_Fr_TMiq
  bus_selector23 : BusSelector  OutputSignals=CAN3_MCUWarn_F
  bus_selector24 : BusSelector  OutputSignals=CAN3_MCU_B_F_RealPwrKw_Sta
  bus_selector3 : BusSelector  OutputSignals=CAN3_Fr_EDURealTMTq
  bus_selector4 : BusSelector  OutputSignals=CAN3_Fr_EDURotateDirction
  bus_selector5 : BusSelector  OutputSignals=CAN3_Fr_EDUTqReqFbk
  bus_selector6 : BusSelector  OutputSignals=CAN3_Fr_MCUBAT
  bus_selector7 : BusSelector  OutputSignals=CAN3_Fr_MCUDCBusCurr
  bus_selector8 : BusSelector  OutputSignals=CAN3_Fr_MCUDCBusVolt
  bus_selector9 : BusSelector  OutputSignals=CAN3_Fr_MCUDischrgSta
  VHAL_FrActvDmpDisabSta_flg : Outport
  VHAL_FrEDUDrtSta_flg : Outport  Port=2
  VHAL_FrEDUOpratingSta_flg : Outport  Port=3
  VHAL_FrEDURealTMTq_Nm : Outport  Port=4
  VHAL_FrEDURotateDirction_enum : Outport  Port=5
  VHAL_FrEDUTqReqFbk_Nm : Outport  Port=6
  VHAL_FrMCUBAT_V : Outport  Port=7
  VHAL_FrMCUDCBusCurr_A : Outport  Port=8
  VHAL_FrMCUDCBusVolt_V : Outport  Port=9
  VHAL_FrMCUDischrgSta_flg : Outport  Port=10
  VHAL_FrMCUEnaSta_flg : Outport  Port=11
  VHAL_FrMCUErr_enum : Outport  Port=12
  VHAL_FrMCUIGNsta_flg : Outport  Port=13
  VHAL_FrMCUReady_flg : Outport  Port=14
  VHAL_FrMCUReady4Pre_flg : Outport  Port=15
  VHAL_FrMCUSysSta_enum : Outport  Port=16
  VHAL_FrMCUTemp_C : Outport  Port=17
  VHAL_FrMotorAvailTq_Nm : Outport  Port=18
  VHAL_FrRegenAvailTq_Nm : Outport  Port=19
  VHAL_FrTMSpd_rpm : Outport  Port=20
  VHAL_FrTMTemp_C : Outport  Port=21
  VHAL_FrTMid_A : Outport  Port=22
  VHAL_FrTMiq_A : Outport  Port=23
  VHAL_MCUWarnF_enum : Outport  Port=24
  VHAL_MCUBFRealPwrKwSta_kW : Outport  Port=25
  wires:
  DT_CAN3_SG_MCU_B_F1/1 -> [DT_CAN3_SG_MCU_B_F1]
  [DT_CAN3_SG_MCU_B_F1] -> bus_selector/1
  bus_selector/1 -> FrActvDmpDisabSta/1(Fr_ActvDmpDisabSta)  "<CAN3_Fr_ActvDmpDisabSta>"
  FrActvDmpDisabSta/1(VHAL_FrActvDmpDisabSta_flg) -> VHAL_FrActvDmpDisabSta_flg/1
  [DT_CAN3_SG_MCU_B_F1] -> bus_selector1/1
  bus_selector1/1 -> FrEDUDrtSta/1(Fr_EDUDrtSta)  "<CAN3_Fr_EDUDrtSta>"
  FrEDUDrtSta/1(VHAL_FrEDUDrtSta_flg) -> VHAL_FrEDUDrtSta_flg/1
  [DT_CAN3_SG_MCU_B_F1] -> bus_selector2/1
  bus_selector2/1 -> FrEDUOpratingSta/1(Fr_EDUOpratingSta)  "<CAN3_Fr_EDUOpratingSta>"
  FrEDUOpratingSta/1(VHAL_FrEDUOpratingSta_flg) -> VHAL_FrEDUOpratingSta_flg/1
  [DT_CAN3_SG_MCU_B_F1] -> bus_selector3/1
  bus_selector3/1 -> FrEDURealTMTq/1(Fr_EDURealTMTq)  "<CAN3_Fr_EDURealTMTq>"
  FrEDURealTMTq/1(VHAL_FrEDURealTMTq_Nm) -> VHAL_FrEDURealTMTq_Nm/1
  [DT_CAN3_SG_MCU_B_F1] -> bus_selector4/1
  bus_selector4/1 -> FrEDURotateDirction/1(Fr_EDURotateDirction)  "<CAN3_Fr_EDURotateDirction>"
  FrEDURotateDirction/1(VHAL_FrEDURotateDirction_enum) -> VHAL_FrEDURotateDirction_enum/1
  [DT_CAN3_SG_MCU_B_F1] -> bus_selector5/1
  bus_selector5/1 -> FrEDUTqReqFbk/1(Fr_EDUTqReqFbk)  "<CAN3_Fr_EDUTqReqFbk>"
  FrEDUTqReqFbk/1(VHAL_FrEDUTqReqFbk_Nm) -> VHAL_FrEDUTqReqFbk_Nm/1
  [DT_CAN3_SG_MCU_B_F1] -> bus_selector6/1
  bus_selector6/1 -> FrMCUBAT/1(Fr_MCUBAT)  "<CAN3_Fr_MCUBAT>"
  FrMCUBAT/1(VHAL_FrMCUBAT_V) -> VHAL_FrMCUBAT_V/1
  [DT_CAN3_SG_MCU_B_F1] -> bus_selector7/1
  bus_selector7/1 -> FrMCUDCBusCurr/1(Fr_MCUDCBusCurr)  "<CAN3_Fr_MCUDCBusCurr>"
  FrMCUDCBusCurr/1(VHAL_FrMCUDCBusCurr_A) -> VHAL_FrMCUDCBusCurr_A/1
  [DT_CAN3_SG_MCU_B_F1] -> bus_selector8/1
  bus_selector8/1 -> FrMCUDCBusVolt/1(Fr_MCUDCBusVolt)  "<CAN3_Fr_MCUDCBusVolt>"
  FrMCUDCBusVolt/1(VHAL_FrMCUDCBusVolt_V) -> VHAL_FrMCUDCBusVolt_V/1
  [DT_CAN3_SG_MCU_B_F1] -> bus_selector9/1
  bus_selector9/1 -> FrMCUDischrgSta/1(Fr_MCUDischrgSta)  "<CAN3_Fr_MCUDischrgSta>"
  FrMCUDischrgSta/1(VHAL_FrMCUDischrgSta_flg) -> VHAL_FrMCUDischrgSta_flg/1
  [DT_CAN3_SG_MCU_B_F1] -> bus_selector10/1
  bus_selector10/1 -> FrMCUEnaSta/1(Fr_MCUEnaSta)  "<CAN3_Fr_MCUEnaSta>"
  FrMCUEnaSta/1(VHAL_FrMCUEnaSta_flg) -> VHAL_FrMCUEnaSta_flg/1
  [DT_CAN3_SG_MCU_B_F1] -> bus_selector11/1
  bus_selector11/1 -> FrMCUErr/1(Fr_MCUErr)  "<CAN3_Fr_MCUErr>"
  FrMCUErr/1(VHAL_FrMCUErr_enum) -> VHAL_FrMCUErr_enum/1
  [DT_CAN3_SG_MCU_B_F1] -> bus_selector12/1
  bus_selector12/1 -> FrMCUIGNsta/1(Fr_MCUIGN_sta)  "<CAN3_Fr_MCUIGN_sta>"
  FrMCUIGNsta/1(VHAL_FrMCUIGNsta_flg) -> VHAL_FrMCUIGNsta_flg/1
  [DT_CAN3_SG_MCU_B_F1] -> bus_selector13/1
  bus_selector13/1 -> FrMCUReady/1(Fr_MCUReady)  "<CAN3_Fr_MCUReady>"
  FrMCUReady/1(VHAL_FrMCUReady_flg) -> VHAL_FrMCUReady_flg/1
  [DT_CAN3_SG_MCU_B_F1] -> bus_selector14/1
  bus_selector14/1 -> FrMCUReady4Pre/1(Fr_MCUReady4Pre)  "<CAN3_Fr_MCUReady4Pre>"
  FrMCUReady4Pre/1(VHAL_FrMCUReady4Pre_flg) -> VHAL_FrMCUReady4Pre_flg/1
  [DT_CAN3_SG_MCU_B_F1] -> bus_selector15/1
  bus_selector15/1 -> FrMCUSysSta/1(Fr_MCUSysSta)  "<CAN3_Fr_MCUSysSta>"
  FrMCUSysSta/1(VHAL_FrMCUSysSta_enum) -> VHAL_FrMCUSysSta_enum/1
  [DT_CAN3_SG_MCU_B_F1] -> bus_selector16/1
  bus_selector16/1 -> FrMCUTemp/1(Fr_MCUTemp)  "<CAN3_Fr_MCUTemp>"
  FrMCUTemp/1(VHAL_FrMCUTemp_C) -> VHAL_FrMCUTemp_C/1
  [DT_CAN3_SG_MCU_B_F1] -> bus_selector17/1
  bus_selector17/1 -> FrMotorAvailTq/1(Fr_MotorAvailTq)  "<CAN3_Fr_MotorAvailTq>"
  FrMotorAvailTq/1(VHAL_FrMotorAvailTq_Nm) -> VHAL_FrMotorAvailTq_Nm/1
  [DT_CAN3_SG_MCU_B_F1] -> bus_selector18/1
  bus_selector18/1 -> FrRegenAvailTq/1(Fr_RegenAvailTq)  "<CAN3_Fr_RegenAvailTq>"
  FrRegenAvailTq/1(VHAL_FrRegenAvailTq_Nm) -> VHAL_FrRegenAvailTq_Nm/1
  [DT_CAN3_SG_MCU_B_F1] -> bus_selector19/1
  bus_selector19/1 -> FrTMSpd/1(Fr_TMSpd)  "<CAN3_Fr_TMSpd>"
  FrTMSpd/1(VHAL_FrTMSpd_rpm) -> VHAL_FrTMSpd_rpm/1
  [DT_CAN3_SG_MCU_B_F1] -> bus_selector20/1
  bus_selector20/1 -> FrTMTemp/1(Fr_TMTemp)  "<CAN3_Fr_TMTemp>"
  FrTMTemp/1(VHAL_FrTMTemp_C) -> VHAL_FrTMTemp_C/1
  [DT_CAN3_SG_MCU_B_F1] -> bus_selector21/1
  bus_selector21/1 -> FrTMid/1(Fr_TMid)  "<CAN3_Fr_TMid>"
  FrTMid/1(VHAL_FrTMid_A) -> VHAL_FrTMid_A/1
  [DT_CAN3_SG_MCU_B_F1] -> bus_selector22/1
  bus_selector22/1 -> FrTMiq/1(Fr_TMiq)  "<CAN3_Fr_TMiq>"
  FrTMiq/1(VHAL_FrTMiq_A) -> VHAL_FrTMiq_A/1
  [DT_CAN3_SG_MCU_B_F1] -> bus_selector23/1
  bus_selector23/1 -> MCUWarnF/1(MCUWarn_F)  "<CAN3_MCUWarn_F>"
  MCUWarnF/1(VHAL_MCUWarnF_enum) -> VHAL_MCUWarnF_enum/1
  [DT_CAN3_SG_MCU_B_F1] -> bus_selector24/1
  bus_selector24/1 -> MCUBFRealPwrKwSta/1(MCU_B_F_RealPwrKw_Sta)  "<CAN3_MCU_B_F_RealPwrKw_Sta>"
  MCUBFRealPwrKwSta/1(VHAL_MCUBFRealPwrKwSta_kW) -> VHAL_MCUBFRealPwrKwSta_kW/1

== system halin/HAL_IN/CAN3/MCU_B_F2 ==
  DT_CAN3_SG_MCU_B_F2 : Inport
  FrCoolanttempReq : Subsystem
  FrFailcode1 : Subsystem
  FrFailcode2 : Subsystem
  FrFailcodehistory1 : Subsystem
  FrFailcodehistory2 : Subsystem
  FrLLCTemp : Subsystem
  FrLLCflowReq : Subsystem
  FrMCUHWVer : Subsystem
  FrMCUSWVer : Subsystem
  FrMCUTempWarn : Subsystem
  FrTMTempWarn : Subsystem
  MCUBFLLCTempWarnSta : Subsystem
  bus_selector : BusSelector  OutputSignals=CAN3_Fr_CoolanttempReq
  bus_selector1 : BusSelector  OutputSignals=CAN3_Fr_Failcode1
  bus_selector10 : BusSelector  OutputSignals=CAN3_Fr_TMTempWarn
  bus_selector11 : BusSelector  OutputSignals=CAN3_MCU_B_F_LLCTempWarn_Sta
  bus_selector2 : BusSelector  OutputSignals=CAN3_Fr_Failcode2
  bus_selector3 : BusSelector  OutputSignals=CAN3_Fr_Failcodehistory1
  bus_selector4 : BusSelector  OutputSignals=CAN3_Fr_Failcodehistory2
  bus_selector5 : BusSelector  OutputSignals=CAN3_Fr_LLCTemp
  bus_selector6 : BusSelector  OutputSignals=CAN3_Fr_LLCflowReq
  bus_selector7 : BusSelector  OutputSignals=CAN3_Fr_MCUTempWarn
  bus_selector8 : BusSelector  OutputSignals=CAN3_Fr_MCU_HW_Ver
  bus_selector9 : BusSelector  OutputSignals=CAN3_Fr_MCU_SW_Ver
  VHAL_FrCoolanttempReq_C : Outport
  VHAL_FrFailcode1_enum : Outport  Port=2
  VHAL_FrFailcode2_enum : Outport  Port=3
  VHAL_FrFailcodehistory1_enum : Outport  Port=4
  VHAL_FrFailcodehistory2_enum : Outport  Port=5
  VHAL_FrLLCTemp_C : Outport  Port=6
  VHAL_FrLLCflowReq_Lpmin : Outport  Port=7
  VHAL_FrMCUTempWarn_enum : Outport  Port=8
  VHAL_FrMCUHWVer_enum : Outport  Port=9
  VHAL_FrMCUSWVer_enum : Outport  Port=10
  VHAL_FrTMTempWarn_enum : Outport  Port=11
  VHAL_MCUBFLLCTempWarnSta_enum : Outport  Port=12
  wires:
  DT_CAN3_SG_MCU_B_F2/1 -> [DT_CAN3_SG_MCU_B_F2]
  [DT_CAN3_SG_MCU_B_F2] -> bus_selector/1
  bus_selector/1 -> FrCoolanttempReq/1(Fr_CoolanttempReq)  "<CAN3_Fr_CoolanttempReq>"
  FrCoolanttempReq/1(VHAL_FrCoolanttempReq_C) -> VHAL_FrCoolanttempReq_C/1
  [DT_CAN3_SG_MCU_B_F2] -> bus_selector1/1
  bus_selector1/1 -> FrFailcode1/1(Fr_Failcode1)  "<CAN3_Fr_Failcode1>"
  FrFailcode1/1(VHAL_FrFailcode1_enum) -> VHAL_FrFailcode1_enum/1
  [DT_CAN3_SG_MCU_B_F2] -> bus_selector2/1
  bus_selector2/1 -> FrFailcode2/1(Fr_Failcode2)  "<CAN3_Fr_Failcode2>"
  FrFailcode2/1(VHAL_FrFailcode2_enum) -> VHAL_FrFailcode2_enum/1
  [DT_CAN3_SG_MCU_B_F2] -> bus_selector3/1
  bus_selector3/1 -> FrFailcodehistory1/1(Fr_Failcodehistory1)  "<CAN3_Fr_Failcodehistory1>"
  FrFailcodehistory1/1(VHAL_FrFailcodehistory1_enum) -> VHAL_FrFailcodehistory1_enum/1
  [DT_CAN3_SG_MCU_B_F2] -> bus_selector4/1
  bus_selector4/1 -> FrFailcodehistory2/1(Fr_Failcodehistory2)  "<CAN3_Fr_Failcodehistory2>"
  FrFailcodehistory2/1(VHAL_FrFailcodehistory2_enum) -> VHAL_FrFailcodehistory2_enum/1
  [DT_CAN3_SG_MCU_B_F2] -> bus_selector5/1
  bus_selector5/1 -> FrLLCTemp/1(Fr_LLCTemp)  "<CAN3_Fr_LLCTemp>"
  FrLLCTemp/1(VHAL_FrLLCTemp_C) -> VHAL_FrLLCTemp_C/1
  [DT_CAN3_SG_MCU_B_F2] -> bus_selector6/1
  bus_selector6/1 -> FrLLCflowReq/1(Fr_LLCflowReq)  "<CAN3_Fr_LLCflowReq>"
  FrLLCflowReq/1(VHAL_FrLLCflowReq_Lpmin) -> VHAL_FrLLCflowReq_Lpmin/1
  [DT_CAN3_SG_MCU_B_F2] -> bus_selector7/1
  bus_selector7/1 -> FrMCUTempWarn/1(Fr_MCUTempWarn)  "<CAN3_Fr_MCUTempWarn>"
  FrMCUTempWarn/1(VHAL_FrMCUTempWarn_enum) -> VHAL_FrMCUTempWarn_enum/1
  [DT_CAN3_SG_MCU_B_F2] -> bus_selector8/1
  bus_selector8/1 -> FrMCUHWVer/1(Fr_MCU_HW_Ver)  "<CAN3_Fr_MCU_HW_Ver>"
  FrMCUHWVer/1(VHAL_FrMCUHWVer_enum) -> VHAL_FrMCUHWVer_enum/1
  [DT_CAN3_SG_MCU_B_F2] -> bus_selector9/1
  bus_selector9/1 -> FrMCUSWVer/1(Fr_MCU_SW_Ver)  "<CAN3_Fr_MCU_SW_Ver>"
  FrMCUSWVer/1(VHAL_FrMCUSWVer_enum) -> VHAL_FrMCUSWVer_enum/1
  [DT_CAN3_SG_MCU_B_F2] -> bus_selector10/1
  bus_selector10/1 -> FrTMTempWarn/1(Fr_TMTempWarn)  "<CAN3_Fr_TMTempWarn>"
  FrTMTempWarn/1(VHAL_FrTMTempWarn_enum) -> VHAL_FrTMTempWarn_enum/1
  [DT_CAN3_SG_MCU_B_F2] -> bus_selector11/1
  bus_selector11/1 -> MCUBFLLCTempWarnSta/1(MCU_B_F_LLCTempWarn_Sta)  "<CAN3_MCU_B_F_LLCTempWarn_Sta>"
  MCUBFLLCTempWarnSta/1(VHAL_MCUBFLLCTempWarnSta_enum) -> VHAL_MCUBFLLCTempWarnSta_enum/1

== system halin/HAL_IN/CAN3/MCU_B_R1 ==
  DT_CAN3_SG_MCU_B_R1 : Inport
  MCUBRRealPwrKwSta : Subsystem
  MCUWarnR : Subsystem
  RrActvDmpDisabSta : Subsystem
  RrEDUDrtSta : Subsystem
  RrEDUOpratingSta : Subsystem
  RrEDURealTMTq : Subsystem
  RrEDURotateDirction : Subsystem
  RrEDUTqReqFbk : Subsystem
  RrMCUBAT : Subsystem
  RrMCUDCBusCurr : Subsystem
  RrMCUDCBusVolt : Subsystem
  RrMCUDischrgSta : Subsystem
  RrMCUEnaSta : Subsystem
  RrMCUErr : Subsystem
  RrMCUIGNsta : Subsystem
  RrMCUReady : Subsystem
  RrMCUReady4Pre : Subsystem
  RrMCUSysSta : Subsystem
  RrMCUTemp : Subsystem
  RrMotorAvailTq : Subsystem
  RrRegenAvailTq : Subsystem
  RrTMSpd : Subsystem
  RrTMTemp : Subsystem
  RrTMid : Subsystem
  RrTMiq : Subsystem
  bus_selector : BusSelector  OutputSignals=CAN3_MCUWarn_R
  bus_selector1 : BusSelector  OutputSignals=CAN3_MCU_B_R_RealPwrKw_Sta
  bus_selector10 : BusSelector  OutputSignals=CAN3_Rr_MCUDCBusVolt
  bus_selector11 : BusSelector  OutputSignals=CAN3_Rr_MCUDischrgSta
  bus_selector12 : BusSelector  OutputSignals=CAN3_Rr_MCUEnaSta
  bus_selector13 : BusSelector  OutputSignals=CAN3_Rr_MCUErr
  bus_selector14 : BusSelector  OutputSignals=CAN3_Rr_MCUIGN_sta
  bus_selector15 : BusSelector  OutputSignals=CAN3_Rr_MCUReady
  bus_selector16 : BusSelector  OutputSignals=CAN3_Rr_MCUReady4Pre
  bus_selector17 : BusSelector  OutputSignals=CAN3_Rr_MCUSysSta
  bus_selector18 : BusSelector  OutputSignals=CAN3_Rr_MCUTemp
  bus_selector19 : BusSelector  OutputSignals=CAN3_Rr_MotorAvailTq
  bus_selector2 : BusSelector  OutputSignals=CAN3_Rr_ActvDmpDisabSta
  bus_selector20 : BusSelector  OutputSignals=CAN3_Rr_RegenAvailTq
  bus_selector21 : BusSelector  OutputSignals=CAN3_Rr_TMSpd
  bus_selector22 : BusSelector  OutputSignals=CAN3_Rr_TMTemp
  bus_selector23 : BusSelector  OutputSignals=CAN3_Rr_TMid
  bus_selector24 : BusSelector  OutputSignals=CAN3_Rr_TMiq
  bus_selector3 : BusSelector  OutputSignals=CAN3_Rr_EDUDrtSta
  bus_selector4 : BusSelector  OutputSignals=CAN3_Rr_EDUOpratingSta
  bus_selector5 : BusSelector  OutputSignals=CAN3_Rr_EDURealTMTq
  bus_selector6 : BusSelector  OutputSignals=CAN3_Rr_EDURotateDirction
  bus_selector7 : BusSelector  OutputSignals=CAN3_Rr_EDUTqReqFbk
  bus_selector8 : BusSelector  OutputSignals=CAN3_Rr_MCUBAT
  bus_selector9 : BusSelector  OutputSignals=CAN3_Rr_MCUDCBusCurr
  VHAL_MCUWarnR_enum : Outport
  VHAL_MCUBRRealPwrKwSta_kW : Outport  Port=2
  VHAL_RrActvDmpDisabSta_flg : Outport  Port=3
  VHAL_RrEDUDrtSta_flg : Outport  Port=4
  VHAL_RrEDUOpratingSta_flg : Outport  Port=5
  VHAL_RrEDURealTMTq_Nm : Outport  Port=6
  VHAL_RrEDURotateDirction_enum : Outport  Port=7
  VHAL_RrEDUTqReqFbk_Nm : Outport  Port=8
  VHAL_RrMCUBAT_V : Outport  Port=9
  VHAL_RrMCUDCBusCurr_A : Outport  Port=10
  VHAL_RrMCUDCBusVolt_V : Outport  Port=11
  VHAL_RrMCUDischrgSta_flg : Outport  Port=12
  VHAL_RrMCUEnaSta_flg : Outport  Port=13
  VHAL_RrMCUErr_enum : Outport  Port=14
  VHAL_RrMCUIGNsta_flg : Outport  Port=15
  VHAL_RrMCUReady_flg : Outport  Port=16
  VHAL_RrMCUReady4Pre_flg : Outport  Port=17
  VHAL_RrMCUSysSta_enum : Outport  Port=18
  VHAL_RrMCUTemp_C : Outport  Port=19
  VHAL_RrMotorAvailTq_Nm : Outport  Port=20
  VHAL_RrRegenAvailTq_Nm : Outport  Port=21
  VHAL_RrTMSpd_rpm : Outport  Port=22
  VHAL_RrTMTemp_C : Outport  Port=23
  VHAL_RrTMid_A : Outport  Port=24
  VHAL_RrTMiq_A : Outport  Port=25
  wires:
  DT_CAN3_SG_MCU_B_R1/1 -> [DT_CAN3_SG_MCU_B_R1]
  [DT_CAN3_SG_MCU_B_R1] -> bus_selector/1
  bus_selector/1 -> MCUWarnR/1(MCUWarn_R)  "<CAN3_MCUWarn_R>"
  MCUWarnR/1(VHAL_MCUWarnR_enum) -> VHAL_MCUWarnR_enum/1
  [DT_CAN3_SG_MCU_B_R1] -> bus_selector1/1
  bus_selector1/1 -> MCUBRRealPwrKwSta/1(MCU_B_R_RealPwrKw_Sta)  "<CAN3_MCU_B_R_RealPwrKw_Sta>"
  MCUBRRealPwrKwSta/1(VHAL_MCUBRRealPwrKwSta_kW) -> VHAL_MCUBRRealPwrKwSta_kW/1
  [DT_CAN3_SG_MCU_B_R1] -> bus_selector2/1
  bus_selector2/1 -> RrActvDmpDisabSta/1(Rr_ActvDmpDisabSta)  "<CAN3_Rr_ActvDmpDisabSta>"
  RrActvDmpDisabSta/1(VHAL_RrActvDmpDisabSta_flg) -> VHAL_RrActvDmpDisabSta_flg/1
  [DT_CAN3_SG_MCU_B_R1] -> bus_selector3/1
  bus_selector3/1 -> RrEDUDrtSta/1(Rr_EDUDrtSta)  "<CAN3_Rr_EDUDrtSta>"
  RrEDUDrtSta/1(VHAL_RrEDUDrtSta_flg) -> VHAL_RrEDUDrtSta_flg/1
  [DT_CAN3_SG_MCU_B_R1] -> bus_selector4/1
  bus_selector4/1 -> RrEDUOpratingSta/1(Rr_EDUOpratingSta)  "<CAN3_Rr_EDUOpratingSta>"
  RrEDUOpratingSta/1(VHAL_RrEDUOpratingSta_flg) -> VHAL_RrEDUOpratingSta_flg/1
  [DT_CAN3_SG_MCU_B_R1] -> bus_selector5/1
  bus_selector5/1 -> RrEDURealTMTq/1(Rr_EDURealTMTq)  "<CAN3_Rr_EDURealTMTq>"
  RrEDURealTMTq/1(VHAL_RrEDURealTMTq_Nm) -> VHAL_RrEDURealTMTq_Nm/1
  [DT_CAN3_SG_MCU_B_R1] -> bus_selector6/1
  bus_selector6/1 -> RrEDURotateDirction/1(Rr_EDURotateDirction)  "<CAN3_Rr_EDURotateDirction>"
  RrEDURotateDirction/1(VHAL_RrEDURotateDirction_enum) -> VHAL_RrEDURotateDirction_enum/1
  [DT_CAN3_SG_MCU_B_R1] -> bus_selector7/1
  bus_selector7/1 -> RrEDUTqReqFbk/1(Rr_EDUTqReqFbk)  "<CAN3_Rr_EDUTqReqFbk>"
  RrEDUTqReqFbk/1(VHAL_RrEDUTqReqFbk_Nm) -> VHAL_RrEDUTqReqFbk_Nm/1
  [DT_CAN3_SG_MCU_B_R1] -> bus_selector8/1
  bus_selector8/1 -> RrMCUBAT/1(Rr_MCUBAT)  "<CAN3_Rr_MCUBAT>"
  RrMCUBAT/1(VHAL_RrMCUBAT_V) -> VHAL_RrMCUBAT_V/1
  [DT_CAN3_SG_MCU_B_R1] -> bus_selector9/1
  bus_selector9/1 -> RrMCUDCBusCurr/1(Rr_MCUDCBusCurr)  "<CAN3_Rr_MCUDCBusCurr>"
  RrMCUDCBusCurr/1(VHAL_RrMCUDCBusCurr_A) -> VHAL_RrMCUDCBusCurr_A/1
  [DT_CAN3_SG_MCU_B_R1] -> bus_selector10/1
  bus_selector10/1 -> RrMCUDCBusVolt/1(Rr_MCUDCBusVolt)  "<CAN3_Rr_MCUDCBusVolt>"
  RrMCUDCBusVolt/1(VHAL_RrMCUDCBusVolt_V) -> VHAL_RrMCUDCBusVolt_V/1
  [DT_CAN3_SG_MCU_B_R1] -> bus_selector11/1
  bus_selector11/1 -> RrMCUDischrgSta/1(Rr_MCUDischrgSta)  "<CAN3_Rr_MCUDischrgSta>"
  RrMCUDischrgSta/1(VHAL_RrMCUDischrgSta_flg) -> VHAL_RrMCUDischrgSta_flg/1
  [DT_CAN3_SG_MCU_B_R1] -> bus_selector12/1
  bus_selector12/1 -> RrMCUEnaSta/1(Rr_MCUEnaSta)  "<CAN3_Rr_MCUEnaSta>"
  RrMCUEnaSta/1(VHAL_RrMCUEnaSta_flg) -> VHAL_RrMCUEnaSta_flg/1
  [DT_CAN3_SG_MCU_B_R1] -> bus_selector13/1
  bus_selector13/1 -> RrMCUErr/1(Rr_MCUErr)  "<CAN3_Rr_MCUErr>"
  RrMCUErr/1(VHAL_RrMCUErr_enum) -> VHAL_RrMCUErr_enum/1
  [DT_CAN3_SG_MCU_B_R1] -> bus_selector14/1
  bus_selector14/1 -> RrMCUIGNsta/1(Rr_MCUIGN_sta)  "<CAN3_Rr_MCUIGN_sta>"
  RrMCUIGNsta/1(VHAL_RrMCUIGNsta_flg) -> VHAL_RrMCUIGNsta_flg/1
  [DT_CAN3_SG_MCU_B_R1] -> bus_selector15/1
  bus_selector15/1 -> RrMCUReady/1(Rr_MCUReady)  "<CAN3_Rr_MCUReady>"
  RrMCUReady/1(VHAL_RrMCUReady_flg) -> VHAL_RrMCUReady_flg/1
  [DT_CAN3_SG_MCU_B_R1] -> bus_selector16/1
  bus_selector16/1 -> RrMCUReady4Pre/1(Rr_MCUReady4Pre)  "<CAN3_Rr_MCUReady4Pre>"
  RrMCUReady4Pre/1(VHAL_RrMCUReady4Pre_flg) -> VHAL_RrMCUReady4Pre_flg/1
  [DT_CAN3_SG_MCU_B_R1] -> bus_selector17/1
  bus_selector17/1 -> RrMCUSysSta/1(Rr_MCUSysSta)  "<CAN3_Rr_MCUSysSta>"
  RrMCUSysSta/1(VHAL_RrMCUSysSta_enum) -> VHAL_RrMCUSysSta_enum/1
  [DT_CAN3_SG_MCU_B_R1] -> bus_selector18/1
  bus_selector18/1 -> RrMCUTemp/1(Rr_MCUTemp)  "<CAN3_Rr_MCUTemp>"
  RrMCUTemp/1(VHAL_RrMCUTemp_C) -> VHAL_RrMCUTemp_C/1
  [DT_CAN3_SG_MCU_B_R1] -> bus_selector19/1
  bus_selector19/1 -> RrMotorAvailTq/1(Rr_MotorAvailTq)  "<CAN3_Rr_MotorAvailTq>"
  RrMotorAvailTq/1(VHAL_RrMotorAvailTq_Nm) -> VHAL_RrMotorAvailTq_Nm/1
  [DT_CAN3_SG_MCU_B_R1] -> bus_selector20/1
  bus_selector20/1 -> RrRegenAvailTq/1(Rr_RegenAvailTq)  "<CAN3_Rr_RegenAvailTq>"
  RrRegenAvailTq/1(VHAL_RrRegenAvailTq_Nm) -> VHAL_RrRegenAvailTq_Nm/1
  [DT_CAN3_SG_MCU_B_R1] -> bus_selector21/1
  bus_selector21/1 -> RrTMSpd/1(Rr_TMSpd)  "<CAN3_Rr_TMSpd>"
  RrTMSpd/1(VHAL_RrTMSpd_rpm) -> VHAL_RrTMSpd_rpm/1
  [DT_CAN3_SG_MCU_B_R1] -> bus_selector22/1
  bus_selector22/1 -> RrTMTemp/1(Rr_TMTemp)  "<CAN3_Rr_TMTemp>"
  RrTMTemp/1(VHAL_RrTMTemp_C) -> VHAL_RrTMTemp_C/1
  [DT_CAN3_SG_MCU_B_R1] -> bus_selector23/1
  bus_selector23/1 -> RrTMid/1(Rr_TMid)  "<CAN3_Rr_TMid>"
  RrTMid/1(VHAL_RrTMid_A) -> VHAL_RrTMid_A/1
  [DT_CAN3_SG_MCU_B_R1] -> bus_selector24/1
  bus_selector24/1 -> RrTMiq/1(Rr_TMiq)  "<CAN3_Rr_TMiq>"
  RrTMiq/1(VHAL_RrTMiq_A) -> VHAL_RrTMiq_A/1
